simulink model "wheel_legged"  (R2023a)
settings: Solver=VariableStepAuto  StartTime=0  StopTime=5  MaxStep=0.05  RelTol=1e-3  AbsTol=1e-3  EnableMultiTasking=on
InitFcn:
  | clc, clear
  | 
  | %Q=diag([800 600 700 1 1000 1]);   %x d_x theta d_theta phi d_phi
  | %R=[1 0;0 0.25];                   %T_A T_B
  | %state_space = load("state_space.mat");
  | %A = state_space.A;
  | %B = state_space.B;
  | %K = lqr(A,B,Q,R);
  | K=test();
  | W_B = 1.3 * 9.81;
  | leg_length = 0.16;
  | thigh = 0.14;
values from neighbouring files (symbols this model uses):
  m = size(B, 2)    [constrainedMPC.m]
  N = 30    [ZOH_discretization.m]    (also in constrainedMPC.m = 20; get_k1_length.m = NM + mp*diff(x + L*sin(theta),t,2))
  X = [x;x_dot;phi;phi_dot;theta_l_1;theta_dot_l_1;theta_l_2;theta_dot_l_2;theta_b;theta_dot_b]    [Newton_Euler_3d.m]
undefined symbols (not defined in the file or in its folder): Y, Z
libraries: sm_lib x24, nesl_utility x15, slpidlib x1
(part 2 of 2)

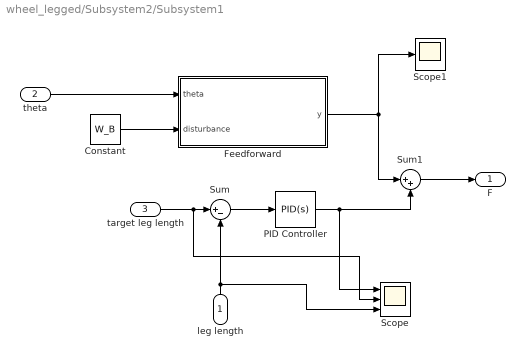
== system wheel_legged/Subsystem2/Subsystem1 ==
  leg length : Inport
  theta : Inport  Port=2
  target leg length : Inport  Port=3
  Constant : Constant  Value=W_B
  Feedforward : MATLAB Function  TreatAsAtomicUnit=on
  PID Controller : slpidlib/PID Controller  Controller=PID  Form=Parallel  TimeDomain=Continuous-time  UseExternalTs=off  SampleTime=-1  IntegratorMethod=Forward Euler  FilterMethod=Forward Euler  ControllerParametersSource=internal  P=200  I=0  UseKiTs=off  D=100  N=100  UseFilter=on  TunerSelectOption=Transfer Function Based (PID Tuner App)  InitialConditionSource=internal  InitialConditionForIntegrator=0  InitialConditionForFilter=0  DifferentiatorICPrevScaledInput=0  ExternalReset=none  TrackingMode=off  Kt=1  LimitOutput=off  SatLimitsSource=internal  UpperSaturationLimit=inf  LowerSaturationLimit=-inf  LinearizeAsGain=on  AntiWindupMode=none  Kb=1  LimitIntegrator=off  UpperIntegratorSaturationLimit=inf  LowerIntegratorSaturationLimit=-inf  POutMin=[]  POutMax=[]  IOutMin=[]  IOutMax=[]  DOutMin=[]  DOutMax=[]  NOutMin=[]  NOutMax=[]  SumOutMin=[]  SumOutMax=[]  SaturationOutMin=[]  SaturationOutMax=[]  PParamMin=[]  PParamMax=[]  IParamMin=[]  IParamMax=[]  DParamMin=[]  DParamMax=[]  NParamMin=[]  NParamMax=[]  KbParamMin=[]  KbParamMax=[]  KtParamMin=[]  KtParamMax=[]  KbOutMin=[]  KbOutMax=[]  KtOutMin=[]  KtOutMax=[]  IntegratorOutMin=[]  IntegratorOutMax=[]  FilterOutMin=[]  FilterOutMax=[]  SumI1OutMin=[]  SumI1OutMax=[]  SumI2OutMin=[]  SumI2OutMax=[]  SumI3OutMin=[]  SumI3OutMax=[]  SumI4OutMin=[]  SumI4OutMax=[]  SumDOutMin=[]  SumDOutMax=[]  DifferentiatorOutMin=[]  DifferentiatorOutMax=[]  FilterDiffOutCoefMin=[]  FilterDiffOutCoefMax=[]  ReciprocalOutMin=[]  ReciprocalOutMax=[]  SumDenOutMin=[]  SumDenOutMax=[]  SumNumOutMin=[]  SumNumOutMax=[]  DivideOutMin=[]  DivideOutMax=[]  UdiffTsProdOutMin=[]  UdiffTsProdOutMax=[]  NTsProdOutMin=[]  NTsProdOutMax=[]  UintegralTsProdOutMin=[]  UintegralTsProdOutMax=[]  UngainTsProdOutMin=[]  UngainTsProdOutMax=[]  ClampingZeroOutDataTypeStr=Inherit: Inherit via back propagation  ClampingZeroOutMin=[]  ClampingZeroOutMax=[]  FilterDenConstantOutDataTypeStr=Inherit: Inherit via back propagation  FilterDenConstantOutMin=[]  FilterDenConstantOutMax=[]  PCopyOutDataTypeStr=Inherit: Inherit via back propagation  PCopyOutMin=[]  PCopyOutMax=[]  NCopyOutDataTypeStr=Inherit: Inherit via back propagation  NCopyOutMin=[]  NCopyOutMax=[]  IntegratorContinuousStateAttributes=''  IntegratorStateMustResolveToSignalObject=off  IntegratorRTWStateStorageClass=Auto  FilterContinuousStateAttributes=''  FilterStateMustResolveToSignalObject=off  FilterRTWStateStorageClass=Auto  ParallelPVariant=InternalParameters  IdealPVariant=Disabled  IVariant=InternalParameters  DVariant=InternalParameters  IntegratorVariant=Continuous  SatVariant=Disabled  AWVariant=Passthrough  PCopyVariant=Disabled  TRVariant=Disabled  FdbkBlocksVariant=Forward  IdealPFdbkVariant=Disabled  SatFdbkVariant=Disabled  DerivativeFilterVariant=ContFilter  NVariant=InternalParameters  NCopyVariant=Disabled  FilterICVariant=InternalICsFilter  IntegratorICVariant=InternalICs  ExternalResetVariant=Disabled  TRSumVariant=Passthrough  SumFdbkVariant=Disabled  SumVariant=Sum_PID  TsampFilterVariant=InternalTs  TsampNgainVariant=Passthrough  TsampIntegralVariant=Disabled_SignalSpec  ExternalSaturationOutDataTypeStr=Inherit: Same as second input
  Scope : Scope  NumInputPorts=3
  Scope1 : Scope
  Sum : Sum  Inputs=|+-
  Sum1 : Sum  Inputs=|++
  F : Outport
  wires:
  leg length/1 -> Scope/3, Sum/2
  target leg length/1 -> Scope/2, Sum/1
  Sum/1 -> PID Controller/1
  theta/1 -> Feedforward/1(theta)
  Feedforward/1(y) -> Scope1/1, Sum1/1
  Sum1/1 -> F/1
  Constant/1 -> Feedforward/2(disturbance)
  PID Controller/1 -> Scope/1, Sum1/2

== matlab function wheel_legged/Subsystem2/MATLAB Function6 ==
  data: F0 input; T1 output; Tp input; phi1 input; phi4 input; T2 output
function [T1,T2] = VMC_calc(F0,Tp,phi1,phi4)

l5=0.16;
l1=0.14;
l2=0.24;
l3=0.24;
l4=0.14;

YD = l4*sin(phi4);
YB = l1*sin(phi1);
XD = l5 + l4*cos(phi4);
XB = l1*cos(phi1); 
lBD = sqrt((XD - XB)*(XD - XB) + (YD - YB)*(YD - YB));
A0 = 2*l2*(XD - XB);
B0 = 2*l2*(YD - YB);
C0 = l2*l2 + lBD*lBD - l3*l3;
phi2 = 2*atan2((B0 + sqrt(A0*A0 + B0*B0 - C0*C0)),A0 + C0);
phi3 = atan2(YB-YD+l2*sin(phi2),XB-XD+l2*cos(phi2));
XC = l1*cos(phi1) + l2*cos(phi2);
YC = l1*sin(phi1) + l2*sin(phi2);
L0 = sqrt((XC - l5/2)*(XC - l5/2) + YC*YC);
phi0 = atan2(YC,XC - l5/2);
j11 = (l1*sin(phi0-phi3)*sin(phi1-phi2))/sin(phi3-phi2);
j12 = (l1*cos(phi0-phi3)*sin(phi1-phi2))/L0*sin(phi3-phi2);
j21 = (l4*sin(phi0-phi2)*sin(phi3-phi4))/sin(phi3-phi2);
j22 = (l4*cos(phi0-phi2)*sin(phi3-phi4))/L0*sin(phi3-phi2);
J = [j11 j12; j21 j22];
F = [F0;Tp];
T = J * F;
T1 = T(1,1);
T2 = T(2,1);

end

== matlab function wheel_legged/MATLAB Function ==
  data: red_pos input; red_position output; red_vel input; green_pos input; green_vel input; red_velocity output; green_position output; green_velocity output
function [red_position, red_velocity, green_position, green_velocity] = coord_trans(red_pos, red_vel, green_pos, green_vel)
    red_position = red_pos + pi;
    green_position = green_pos - pi;
    red_velocity = red_vel;
    green_velocity = green_vel;
end

== matlab function wheel_legged/MATLAB Function1 ==
  data: phi input; phi_dot input; phi_1 input; phi_1_dot input; phi_1 output; phi_4 input; phi_4_dot input; phi_2 output; phi_3 output; phi_4 output; phi_0 output; theta output; theta_dot output; leg_length output; x output; x_dot output; toe_pos input; toe_vel input; phi output; phi_dot output; phi0_dot_new output; x1 output; xe output; y1 output; ye output
function [phi_1, phi_2, phi_3, phi_4, phi_0, theta, theta_dot, leg_length, x, x_dot, phi, phi_dot, phi0_dot_new, x1, xe, y1, ye] = forward_kinematics(phi, phi_dot, phi_1, phi_1_dot, phi_4, phi_4_dot, toe_pos, toe_vel)
thigh_distance = 0.07;
thigh = 0.14;
calf = 0.24;
wheel_radius = 0.03;

x_A = -thigh_distance / 2;
y_A = 0;
x_E = thigh_distance / 2;
y_E = 0;
x_B = x_A + thigh * cos(phi_1);
y_B = y_A + thigh * sin(phi_1);
x_D = x_E + thigh * cos(phi_4);
y_D = y_E + thigh * sin(phi_4);
l_BD_square = (x_B - x_D)^2 + (y_B - y_D)^2;

lyd = 2*calf*y_D;
lyb = 2*calf*y_B;
lxd = 2*calf*x_D;
lxb = 2*calf*x_B;
Y_1 = lyd - lyb + sqrt(-l_BD_square * (-4*calf^2+l_BD_square));

phi_2 = 2 * atan2(Y_1, l_BD_square - lxb + lxd);
phi_3 = mod(-2 * atan2(Y_1, l_BD_square + lxb - lxd), 2*pi);

x_C = x_B + calf * cos(phi_2);
y_C = y_B + calf * sin(phi_2);
phi_0 = (atan2(y_C, x_C));
leg_length = sqrt(x_C^2 + y_C^2);

% theta_dot calculation
x_B_dot = -thigh * phi_1_dot * sin(phi_1);
y_B_dot = thigh * phi_1_dot * cos(phi_1);
x_D_dot = -thigh * phi_1_dot * sin(phi_4);
y_D_dot = thigh * phi_1_dot * cos(phi_4);

% phi_2_dot
%phi_2_dot = ((x_B_dot - x_D_dot) * cos(phi_3) + (y_B_dot - y_D_dot) * sin(phi_3)) / (calf * sin(phi_2 - phi_3));

%x_c_dot = -thigh * phi_1_dot * sin(phi_1) - calf * phi_2_dot * sin(phi_2);
%y_c_dot = thigh * phi_1_dot * cos(phi_1) + calf * phi_2_dot * cos(phi_2);
theta = phi + phi_0 - pi/2;%-(y_c_dot/x_C - (x_c_dot * y_C)/(x_C^2))/((y_C/x_C)^2+1);
l5 = leg_length;
%phi0_dot = ;
% (phi_1_dot*((thigh*cos(phi_1) + (2*calf*cos(2*atan(((4*calf^2*(thigh*sin(phi_1) - thigh*sin(phi_4))^2 - ((thigh*sin(phi_1) - thigh*sin(phi_4))^2 + (l5 - thigh*cos(phi_1) + thigh*cos(phi_4))^2 + calf^2 - calf^2)^2 + 4*calf^2*(l5 - thigh*cos(phi_1) ...
% + thigh*cos(phi_4))^2)^(1/2) - 2*calf*(thigh*sin(phi_1) - thigh*sin(phi_4)))/((thigh*sin(phi_1) - thigh*sin(phi_4))^2 + (l5 - thigh*cos(phi_1) + thigh*cos(phi_4))^2 + calf^2 - calf^2 + 2*calf*(l5 - thigh*cos(phi_1) + thigh*cos(phi_4)))))*(((8*thigh*calf^2*cos(phi_1)*(thigh*sin(phi_1) - thigh*sin(phi_4)) - 2*(2*thigh*cos(phi_1)*(thigh*sin(phi_1) - thigh*sin(phi_4)) + 2*thigh*sin(phi_1)*(l5 - thigh*cos(phi_1) + thigh*cos(phi_4)))*((thigh*sin(phi_1) - thigh*sin(phi_4))^2 + (l5 - thigh*cos(phi_1) + thigh*cos(phi_4))^2 + calf^2 - calf^2) + 8*thigh*calf^2*sin(phi_1)*(l5 - thigh*cos(phi_1) + thigh*cos(phi_4)))/(2*(4*calf^2*(thigh*sin(phi_1) - thigh*sin(phi_4))^2 - ((thigh*sin(phi_1) - thigh*sin(phi_4))^2 + (l5 - thigh*cos(phi_1) + thigh*cos(phi_4))^2 + calf^2 - calf^2)^2 + 4*calf^2*(l5 - thigh*cos(phi_1) + thigh*cos(phi_4))^2)^(1/2)) - 2*thigh*calf*cos(phi_1))/((thigh*sin(phi_1) - thigh*sin(phi_4))^2 + (l5 - thigh*cos(phi_1) + thigh*cos(phi_4))^2 + calf^2 - calf^2 + 2*calf*(l5 - thigh*cos(phi_1) + thigh*cos(phi_4))) - (((4*calf^2*(thigh*sin(phi_1) - thigh*sin(phi_4))^2 - ((thigh*sin(phi_1) - thigh*sin(phi_4))^2 + (l5 - thigh*cos(phi_1) + thigh*cos(phi_4))^2 + calf^2 - calf^2)^2 + 4*calf^2*(l5 - thigh*cos(phi_1) + thigh*cos(phi_4))^2)^(1/2) - 2*calf*(thigh*sin(phi_1) - thigh*sin(phi_4)))*(2*thigh*calf*sin(phi_1) +...
% 2*thigh*cos(phi_1)*(thigh*sin(phi_1) - thigh*sin(phi_4)) + 2*thigh*sin(phi_1)*(l5 - thigh*cos(phi_1) + thigh*cos(phi_4))))/((thigh*sin(phi_1) - thigh*sin(phi_4))^2 + (l5 - thigh*cos(phi_1) + thigh*cos(phi_4))^2 + calf^2 - calf^2 + 2*calf*(l5 - thigh*cos(phi_1) + thigh*cos(phi_4)))^2))/(((4*calf^2*(thigh*sin(phi_1) - thigh*sin(phi_4))^2 - ((thigh*sin(phi_1) - thigh*sin(phi_4))^2 + (l5 - thigh*cos(phi_1) + thigh*cos(phi_4))^2 + calf^2 - calf^2)^2 + 4*calf^2*(l5 - thigh*cos(phi_1) + thigh*cos(phi_4))^2)^(1/2) - 2*calf*(thigh*sin(phi_1) - thigh*sin(phi_4)))^2/((thigh*sin(phi_1) - thigh*sin(phi_4))^2 + (l5 - thigh*cos(phi_1) + thigh*cos(phi_4))^2 + calf^2 - calf^2 + 2*calf*(l5 - thigh*cos(phi_1) + thigh*cos(phi_4)))^2 + 1))/(calf*cos(2*atan(((4*calf^2*(thigh*sin(phi_1) - thigh*sin(phi_4))^2 - ((thigh*sin(phi_1) - thigh*sin(phi_4))^2 + (l5 - thigh*cos(phi_1) + thigh*cos(phi_4))^2 + calf^2 - calf^2)^2 + 4*calf^2*(l5 - thigh*cos(phi_1) + thigh*cos(phi_4))^2)^(1/2) - 2*calf*(thigh*sin(phi_1) - thigh*sin(phi_4)))/((thigh*sin(phi_1) - thigh*sin(phi_4))^2 + (l5 - thigh*cos(phi_1) + thigh*cos(phi_4))^2 + calf^2 - calf^2 + 2*calf*(l5 - thigh*cos(phi_1) + thigh*cos(phi_4))))) - l5/2 + thigh*cos(phi_1)) + ((calf*sin(2*atan(((4*calf^2*(thigh*sin(phi_1) - thigh*sin(phi_4))^2 - ((thigh*sin(phi_1) - thigh*sin(phi_4))^2 + (l5 - thigh*cos(phi_1) + thigh*cos(phi_4))^2 + calf^2 - calf^2)^2 + 4*calf^2*(l5 - thigh*cos(phi_1) + thigh*cos(phi_4))^2)^(1/2) - 2*calf*(thigh*sin(phi_1) - thigh*sin(phi_4)))/((thigh*sin(phi_1) - thigh*sin(phi_4))^2 + (l5 - thigh*cos(phi_1) + thigh*cos(phi_4))^2 + calf^2 - calf^2 + 2*calf*(l5 - thigh*cos(phi_1) + thigh*cos(phi_4))))) + thigh*sin(phi_1))*(thigh*sin(phi_1) + (2*calf*sin(2*atan(((4*calf^2*(thigh*sin(phi_1) - thigh*sin(phi_4))^2 - ((thigh*sin(phi_1) - thigh*sin(phi_4))^2 + (l5 - thigh*cos(phi_1) + thigh*cos(phi_4))^2 + calf^2 - calf^2)^2 + 4*calf^2*(l5 - thigh*cos(phi_1) + thigh*cos(phi_4))^2)^(1/2) - 2*calf*(thigh*sin(phi_1) - thigh*sin(phi_4)))/((thigh*sin(phi_1) - thigh*sin(phi_4))^2 + (l5 - thigh*cos(phi_1) + thigh*cos(phi_4))^2 + calf^2 - calf^2 + 2*calf*(l5 - thigh*cos(phi_1) + thigh*cos(phi_4)))))*(((8*thigh*calf^2*cos(phi_1)*(thigh*sin(phi_1) - thigh*sin(phi_4)) - 2*(2*thigh*cos(phi_1)*(thigh*sin(phi_1) - thigh*sin(phi_4)) + 2*thigh*sin(phi_1)*(l5 - thigh*cos(phi_1) + thigh*cos(phi_4)))*((thigh*sin(phi_1) - thigh*sin(phi_4))^2 + (l5 - thigh*cos(phi_1) + thigh*cos(phi_4))^2 + calf^2 - calf^2) + 8*thigh*calf^2*sin(phi_1)*(l5 - thigh*cos(phi_1) + thigh*cos(phi_4))...
% )/(2*(4*calf^2*(thigh*sin(phi_1) - thigh*sin(phi_4))^2 - ((thigh*sin(phi_1) - thigh*sin(phi_4))^2 + (l5 - thigh*cos(phi_1) + thigh*cos(phi_4))^2 + calf^2 - calf^2)^2 + 4*calf^2*(l5 - thigh*cos(phi_1) + thigh*cos(phi_4))^2)^(1/2)) - 2*thigh*calf*cos(phi_1))/((thigh*sin(phi_1) - thigh*sin(phi_4))^2 + (l5 - thigh*cos(phi_1) + thigh*cos(phi_4))^2 + calf^2 - calf^2 + 2*calf*(l5 - thigh*cos(phi_1) + thigh*cos(phi_4))) - (((4*calf^2*(thigh*sin(phi_1) - thigh*sin(phi_4))^2 - ((thigh*sin(phi_1) - thigh*sin(phi_4))^2 + (l5 - thigh*cos(phi_1) + thigh*cos(phi_4))^2 + calf^2 - calf^2)^2 + 4*calf^2*(l5 - thigh*cos(phi_1) + thigh*cos(phi_4))^2)^(1/2) - 2*calf*(thigh*sin(phi_1) - thigh*sin(phi_4)))*(2*thigh*calf*sin(phi_1) + 2*thigh*cos(phi_1)*(thigh*sin(phi_1) - thigh*sin(phi_4)) + 2*thigh*sin(phi_1)*(l5 - thigh*cos(phi_1) + thigh*cos(phi_4))))/((thigh*sin(phi_1) - thigh*sin(phi_4))^2 + (l5 - thigh*cos(phi_1) + thigh*cos(phi_4))^2 + calf^2 - calf^2 + 2*calf*(l5 - thigh*cos(phi_1) + thigh*cos(phi_4)))^2))/(((4*calf^2*(thigh*sin(phi_1) - thigh*sin(phi_4))^2 - ((thigh*sin(phi_1) - thigh*sin(phi_4))^2 + (l5 - thigh*cos(phi_1) + thigh*cos(phi_4))^2 + calf^2 - calf^2)^2 + 4*calf^2*(l5 - thigh*cos(phi_1) + thigh*cos(phi_4))^2)^(1/2) - 2*calf*(thigh*sin(phi_1) - thigh*sin(phi_4)))^2/((thigh*sin(phi_1) - thigh*sin(phi_4))^2 + (l5 - thigh*cos(phi_1) + thigh*cos(phi_4))^2 + calf^2 - calf^2 + 2*calf*(l5 - thigh*cos(phi_1) + thigh*cos(phi_4)))^2 + 1)))/(calf*cos(2*atan(((4*calf^2*(thigh*sin(phi_1) - thigh*sin(phi_4))^2 - ((thigh*sin(phi_1) - thigh*sin(phi_4))^2 + (l5 - thigh*cos(phi_1) + thigh*cos(phi_4))^2 + calf^2 - calf^2)^2 + 4*calf^2*(l5 - thigh*cos(phi_1) + thigh*cos(phi_4))^2)^(1/2) - 2*calf*(thigh*sin(phi_1) - thigh*sin(phi_4)))/((thigh*sin(phi_1) - thigh*sin(phi_4))^2 + (l5 - thigh*cos(phi_1) + thigh*cos(phi_4))^2 + calf^2 - calf^2 + 2*calf*(l5 - thigh*cos(phi_1) + thigh*cos(phi_4))))) - l5/2 + thigh*cos(phi_1))^2))/((calf*sin(2*atan(((4*calf^2*(thigh*sin(phi_1) - thigh*sin(phi_4))^2 - ((thigh*sin(phi_1) - thigh*sin(phi_4))^2 + (l5 - thigh*cos(phi_1) + thigh*cos(phi_4))^2 + calf^2 - calf^2)^2 + 4*calf^2*(l5 - thigh*cos(phi_1) + thigh*cos(phi_4))^2)^(1/2) - 2*calf*(thigh*sin(phi_1) - thigh*sin(phi_4)))/((thigh*sin(phi_1) - thigh*sin(phi_4))^2 + (l5 - thigh*cos(phi_1) + thigh*cos(phi_4))^2 + calf^2 - calf^2 + 2*calf*(l5 - thigh*cos(phi_1) + thigh*cos(phi_4))))) + thigh*sin(phi_1))^2/(calf*cos(2*atan(((4*calf^2*(thigh*sin(phi_1) - thigh*sin(phi_4))^2 - ((thigh*sin(phi_1) - thigh*sin(phi_4))^2 + (l5 - thigh*cos(phi_1) + thigh*cos(phi_4))^2 + calf^2 - calf^2)^2 + 4*calf^2*(l5 - thigh*cos(phi_1) + thigh*cos(phi_4))^2)^(1/2) - 2*calf*(thigh*sin(phi_1) - thigh*sin(phi_4)))/((thigh*sin(phi_1) - thigh*sin(phi_4))^2 + (l5 - thigh*cos(phi_1) + thigh*cos(phi_4))^2 + calf^2 - calf^2 + 2*calf*(l5 - thigh*cos(phi_1) + thigh*cos(phi_4))))) - l5/2 + thigh*cos(phi_1))^2 + 1) - (phi_4_dot*((2*calf*cos(2*atan(((4*calf^2*(thigh*sin(phi_1) - thigh*sin(phi_4))^2 - ((thigh*sin(phi_1) - thigh*sin(phi_4))^2 + (l5 - thigh*cos(phi_1) + thigh*cos(phi_4))^2 + calf^2 - calf^2)^2 + 4*calf^2*(l5 - thigh*cos(phi_1) + thigh*cos(phi_4))^2)^(1/2) - 2*calf*(thigh*sin(phi_1) - thigh*sin(phi_4)))/((thigh*sin(phi_1) - thigh*sin(phi_4))^2 + (l5 - thigh*cos(phi_1) + thigh*cos(phi_4))^2 + calf^2 - calf^2 + 2*calf*(l5 - thigh*cos(phi_1) + thigh*cos(phi_4)))))*(((8*calf^2*thigh*cos(phi_4)*(thigh*sin(phi_1) - thigh*sin(phi_4)) - 2*(2*thigh*cos(phi_4)*(thigh*sin(phi_1) - thigh*sin(phi_4)) + 2*thigh*sin(phi_4)*(l5 - thigh*cos(phi_1) + thigh*cos(phi_4)))*((thigh*sin(phi_1) - thigh*sin(phi_4))^2 + (l5 - thigh*cos(phi_1) + thigh*cos(phi_4))^2 + calf^2 - calf^2) + 8*calf^2*thigh*sin(phi_4)*(l5 - thigh*cos(phi_1) + thigh*cos(phi_4)))/(2*(4*calf^2*(thigh*sin(phi_1) - thigh*sin(phi_4))^2 - ((thigh*sin(phi_1) - thigh*sin(phi_4))^2 + (l5 - thigh*cos(phi_1) + thigh*cos(phi_4))^2 + calf^2 - calf^2)^2 + 4*calf^2*(l5 - thigh*cos(phi_1) + thigh*cos(phi_4))^2)^(1/2)) - 2*calf*thigh*cos(phi_4))/((thigh*sin(phi_1) - thigh*sin(phi_4))^2 + (l5 - thigh*cos(phi_1) + thigh*cos(phi_4))^2 + calf^2 - calf^2 + 2*calf*(l5 - thigh*cos(phi_1) + thigh*cos(phi_4))) - (((4*calf^2*(thigh*sin(phi_1) - thigh*sin(phi_4))^2 - ((thigh*sin(phi_1) - thigh*sin(phi_4))^2 + (l5 - thigh*cos(phi_1) + thigh*cos(phi_4))^2 + calf^2 - calf^2)^2 + 4*calf^2*(l5 - thigh*cos(phi_1) + thigh*cos(phi_4))^2)^(1/2) - 2*calf*(thigh*sin(phi_1) - thigh*sin(phi_4)))*(2*calf*thigh*sin(phi_4) + 2*thigh*cos(phi_4)*(thigh*sin(phi_1) - thigh*sin(phi_4)) + 2*thigh*sin(phi_4)*(l5 - thigh*cos(phi_1) + thigh*cos(phi_4))))/((thigh*sin(phi_1) - thigh*sin(phi_4))^2 + (l5 - thigh*cos(phi_1) + thigh*cos(phi_4))^2 + calf^2 - calf^2 + 2*calf*(l5 - thigh*cos(phi_1) + thigh*cos(phi_4)))^2))/((((4*calf^2*(thigh*sin(phi_1) - thigh*sin(phi_4))^2 - ((thigh*sin(phi_1) - thigh*sin(phi_4))^2 + (l5 - thigh*cos(phi_1) + thigh*cos(phi_4))^2 + calf^2 - calf^2)^2 + 4*calf^2*(l5 - thigh*cos(phi_1) + thigh*cos(phi_4))^2)^(1/2) - 2*calf*(thigh*sin(phi_1) - thigh*sin(phi_4)))^2/((thigh*sin(phi_1) - thigh*sin(phi_4))^2 + (l5 - thigh*cos(phi_1) + thigh*cos(phi_4))^2 + calf^2 - calf^2 + 2*calf*(l5 - thigh*cos(phi_1) + thigh*cos(phi_4)))^2 + 1)*(calf*cos(2*atan(((4*calf^2*(thigh*sin(phi_1) - thigh*sin(phi_4))^2 - ((thigh*sin(phi_1) - thigh*sin(phi_4))^2 + (l5 - thigh*cos(phi_1) + thigh*cos(phi_4))^2 + calf^2 - calf^2)^2 + 4*calf^2*(l5 - thigh*cos(phi_1) + thigh*cos(phi_4))^2)^(1/2) - 2*calf*(thigh*sin(phi_1) - thigh*sin(phi_4)))/((thigh*sin(phi_1) - thigh*sin(phi_4))^2 + (l5 - thigh*cos(phi_1) + thigh*cos(phi_4))^2 + calf^2 - calf^2 + 2*calf*(l5 - thigh*cos(phi_1) + thigh*cos(phi_4))))) - l5/2 + thigh*cos(phi_1))) + (2*calf*sin(2*atan(((4*calf^2*(thigh*sin(phi_1) - thigh*sin(phi_4))^2 - ((thigh*sin(phi_1) - thigh*sin(phi_4))^2 + (l5 - thigh*cos(phi_1) + thigh*cos(phi_4))^2 + calf^2 - calf^2)^2 + 4*calf^2*(l5 - thigh*cos(phi_1) + thigh*cos(phi_4))^2)^(1/2) - 2*calf*(thigh*sin(phi_1) - thigh*sin(phi_4)))/((thigh*sin(phi_1) - thigh*sin(phi_4))^2 + (l5 - thigh*cos(phi_1) + thigh*cos(phi_4))^2 + calf^2 - calf^2 + 2*calf*(l5 - thigh*cos(phi_1) + thigh*cos(phi_4)))))*(calf*sin(2*atan(((4*calf^2*(thigh*sin(phi_1) - thigh*sin(phi_4))^2 - ((thigh*sin(phi_1) - thigh*sin(phi_4))^2 + (l5 - thigh*cos(phi_1) + thigh*cos(phi_4))^2 + calf^2 - calf^2)^2 + 4*calf^2*(l5 - thigh*cos(phi_1) + thigh*cos(phi_4))^2)^(1/2) - 2*calf*(thigh*sin(phi_1) - thigh*sin(phi_4)))/((thigh*sin(phi_1) - thigh*sin(phi_4))^2 + (l5 - thigh*cos(phi_1) + thigh*cos(phi_4))^2 + calf^2 - calf^2 + 2*calf*(l5 - thigh*cos(phi_1) + thigh*cos(phi_4))))) + thigh*sin(phi_1))*(((8*calf^2*thigh*cos(phi_4)*(thigh*sin(phi_1) - thigh*sin(phi_4)) - 2*(2*thigh*cos(phi_4)*(thigh*sin(phi_1) - thigh*sin(phi_4)) + 2*thigh*sin(phi_4)*(l5 - thigh*cos(phi_1) + thigh*cos(phi_4)))*((thigh*sin(phi_1) - thigh*sin(phi_4))^2 + (l5 - thigh*cos(phi_1) + thigh*cos(phi_4))^2 + calf^2 - calf^2) + 8*calf^2*thigh*sin(phi_4)*(l5 - thigh*cos(phi_1) + thigh*cos(phi_4)))/(2*(4*calf^2*(thigh*sin(phi_1) - thigh*sin(phi_4))^2 - ((thigh*sin(phi_1) - thigh*sin(phi_4))^2 + (l5 - thigh*cos(phi_1) + thigh*cos(phi_4))^2 + calf^2 - calf^2)^2 + 4*calf^2*(l5 - thigh*cos(phi_1) + thigh*cos(phi_4))^2)^(1/2)) - 2*calf*thigh*cos(phi_4))/((thigh*sin(phi_1) - thigh*sin(phi_4))^2 + (l5 - thigh*cos(phi_1) + thigh*cos(phi_4))^2 + calf^2 - calf^2 + 2*calf*(l5 - thigh*cos(phi_1) + thigh*cos(phi_4))) - (((4*calf^2*(thigh*sin(phi_1) - thigh*sin(phi_4))^2 - ((thigh*sin(phi_1) - thigh*sin(phi_4))^2 + (l5 - thigh*cos(phi_1) + thigh*cos(phi_4))^2 + calf^2 - calf^2)^2 + 4*calf^2*(l5 - thigh*cos(phi_1) + thigh*cos(phi_4))^2)^(1/2) - 2*calf*(thigh*sin(phi_1) - thigh*sin(phi_4)))*(2*calf*thigh*sin(phi_4) + 2*thigh*cos(phi_4)*(thigh*sin(phi_1) - thigh*sin(phi_4)) + 2*thigh*sin(phi_4)*(l5 - thigh*cos(phi_1) + thigh*cos(phi_4))))/((thigh*sin(phi_1) - thigh*sin(phi_4))^2 + (l5 - thigh*cos(phi_1) + thigh*cos(phi_4))^2 + calf^2 - calf^2 + 2*calf*(l5 - thigh*cos(phi_1) + thigh*cos(phi_4)))^2))/((((4*calf^2*(thigh*sin(phi_1) - thigh*sin(phi_4))^2 - ((thigh*sin(phi_1) - thigh*sin(phi_4))^2 + (l5 - thigh*cos(phi_1) + thigh*cos(phi_4))^2 + calf^2 - calf^2)^2 + 4*calf^2*(l5 - thigh*cos(phi_1) + thigh*cos(phi_4))^2)^(1/2) - 2*calf*(thigh*sin(phi_1) - thigh*sin(phi_4)))^2/((thigh*sin(phi_1) - thigh*sin(phi_4))^2 + (l5 - thigh*cos(phi_1) + thigh*cos(phi_4))^2 + calf^2 - calf^2 + 2*calf*(l5 - thigh*cos(phi_1) + thigh*cos(phi_4)))^2 + 1)*(calf*cos(2*atan(((4*calf^2*(thigh*sin(phi_1) - thigh*sin(phi_4))^2 - ((thigh*sin(phi_1) - thigh*sin(phi_4))^2 + (l5 - thigh*cos(phi_1) + thigh*cos(phi_4))^2 + calf^2 - calf^2)^2 + 4*calf^2*(l5 - thigh*cos(phi_1) + thigh*cos(phi_4))^2)^(1/2) - 2*calf*(thigh*sin(phi_1) - thigh*sin(phi_4)))/((thigh*sin(phi_1) - thigh*sin(phi_4))^2 + (l5 - thigh*cos(phi_1) + thigh*cos(phi_4))^2 + calf^2 - calf^2 + 2*calf*(l5 - thigh*cos(phi_1) + thigh*cos(phi_4))))) - l5/2 + thigh*cos(phi_1))^2)))/((calf*sin(2*atan(((4*calf^2*(thigh*sin(phi_1) - thigh*sin(phi_4))^2 - ((thigh*sin(phi_1) - thigh*sin(phi_4))^2 + (l5 - thigh*cos(phi_1) + thigh*cos(phi_4))^2 + calf^2 - calf^2)^2 + 4*calf^2*(l5 - thigh*cos(phi_1) + thigh*cos(phi_4))^2)^(1/2) - 2*calf*(thigh*sin(phi_1) - thigh*sin(phi_4)))/((thigh*sin(phi_1) - thigh*sin(phi_4))^2 + (l5 - thigh*cos(phi_1) + thigh*cos(phi_4))^2 + calf^2 - calf^2 + 2*calf*(l5 - thigh*cos(phi_1) + thigh*cos(phi_4))))) + thigh*sin(phi_1))^2/(calf*cos(2*atan(((4*calf^2*(thigh*sin(phi_1) - thigh*sin(phi_4))^2 - ((thigh*sin(phi_1) - thigh*sin(phi_4))^2 + (l5 - thigh*cos(phi_1) + thigh*cos(phi_4))^2 + calf^2 - calf^2)^2 + 4*calf^2*(l5 - thigh*cos(phi_1) + thigh*cos(phi_4))^2)^(1/2) - 2*calf*(thigh*sin(phi_1) - thigh*sin(phi_4)))/((thigh*sin(phi_1) - thigh*sin(phi_4))^2 + (l5 - thigh*cos(phi_1) + thigh*cos(phi_4))^2 + calf^2 - calf^2 + 2*calf*(l5 - thigh*cos(phi_1) + thigh*cos(phi_4))))) - l5/2 + thigh*cos(phi_1))^2 + 1);

%theta_dot = phi_dot + phi0_dot;
x1 = thigh - calf * cos(phi_1);
xe = -x_C;
y1 = calf * sin(phi_1);
ye = y_C;

l = l5;
numerator = phi_1_dot * calf * (sin(phi_1) * (x1-xe) + cos(phi_1) * (ye-y1));
dominator = - l*(cos(phi_0 - pi/2)*(x1-xe)+sin(phi_0 - pi/2)*(ye-y1));
phi0_dot_new = numerator/dominator;
theta_dot = phi_dot + phi0_dot_new;
% x
x = -toe_pos * wheel_radius;
x_dot = -toe_vel * wheel_radius;
end

== matlab function wheel_legged/Subsystem2/Subsystem1/Feedforward ==
  data: theta input; y output; disturbance input
function y = fcn(theta, disturbance)

y = disturbance / cos(theta);

== matlab function wheel_legged/Subsystem2/MATLAB Function2 ==
  data: T_B input; T_1 output; F input; leg_length input; theta input; T_4 output; phi1 input; phi2 input; phi3 input; phi4 input
function [T_1, T_4]= vmc(T_B, F, leg_length, theta, phi1, phi2, phi3, phi4)
thigh = 0.14;
theta = pi/2 + theta;
j11 = thigh * sin(theta - phi3) * sin(phi1 - phi2) / sin(phi3 - phi2);
j12 = thigh * cos(theta - phi3) * sin(phi1 - phi2) / (leg_length * sin(phi3 - phi2));
j21 = thigh * sin(theta - phi2) * sin(phi3 - phi4) / sin(phi3 - phi2);
j22 = thigh * cos(theta - phi2) * sin(phi3 - phi4) / (leg_length * sin(phi3 - phi2));
J = [j11 j12;
     j21 j22];

T = J * [F;T_B];
T_1 = T(1);
T_4 = T(2);
end
